simulink model "fletcher_gen"  (R2014b)
settings: Solver=ode45  StartTime=0.0  StopTime=10.0  RelTol=1e-3
settings Model: Creator=Ben Windo  LastModifiedBy=Ben Windo
settings DataIOCC: ExternalInput=[(t),(2)]; t=(0:2);  LoadExternalInput=on

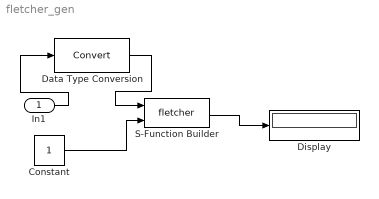
== system fletcher_gen ==
  In1 : Inport  OutDataTypeStr=double
  Constant : Constant
  Data Type Conversion : DataTypeConversion
  Display : Display
  S-Function Builder : S-Function  InitFcn=try, set_param(gcb,'FunctionName','fletcher'), end  FunctionName=fletcher  SFunctionModules=fletcher_wrapper  EnableBusSupport=off  mask(S-Function Builder){}
      mask help: Simulink:masks:SFunctionBuilder_MD
      mask init:
      | val = [[.9  0.75 0.75 1 1 .9 .9 1]',[1 1 0.75 0.75 .9 .9 1 .9]'];try , sys = get_param(gcb,'SfunBuilderFcnName');if isempty(sys), sys = get_param(gcb,'FunctionName'); end,catch, sys = get_param(gcb,'FunctionName'); end
      settings: CopyFcn=set_param(gcbh,'LinkStatus','none')  PreSaveFcn=try, set_param(gcb,'FunctionName','fletcher'), end  OpenFcn=sfunctionwizard(gcbh)
      mask Display: plot(val(:,1),val(:,2)),disp(sys), port_label('input',1,'u0'), port_label('input',2,'count'), port_label('output',1,'y0')
  wires:
  Constant/1 -> S-Function Builder/2
  S-Function Builder/1 -> Display/1
  Data Type Conversion/1 -> S-Function Builder/1
  In1/1 -> Data Type Conversion/1
